simulink model "test"  (R2021a)
settings: Solver=ode4  StartTime=0.0  StopTime=0.001  FixedStep=1e-3  RelTol=1e-3
settings Model: Creator=valeriytashchilin  LastModifiedBy=valeriytashchilin
settings DataIOCC: SaveFinalState=on  SaveFormat=Array  SaveState=on

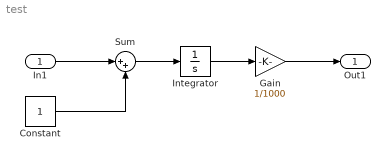
== system test ==
  In1 : Inport
  Constant : Constant
  Gain : Gain  Gain=1/1000
  Integrator : Integrator
  Sum : Sum  Inputs=|++
  Out1 : Outport
  wires:
  In1/1 -> Sum/1
  Constant/1 -> Sum/2
  Sum/1 -> Integrator/1
  Integrator/1 -> Gain/1
  Gain/1 -> Out1/1
